simulink model "HeadingControl_DiffDriveRover"  (R2021a)
settings: Solver=ode45  StartTime=0.0  StopTime=15  RelTol=1e-3
values from neighbouring files (symbols this model uses):
  den_motor = [J*L, (J*R + b*L), (b*R + K^2)]    [heading_control_rover.m]
  Kd = 0.8    [heading_control_rover.m]
  Ki = 1.5    [heading_control_rover.m]
  Kp = 5.0    (= 5)    [heading_control_rover.m]
  L_base = 0.30    (= 0.3)    [heading_control_rover.m]
  num_motor = [K]    [heading_control_rover.m]
  r_wheel = 0.05    [heading_control_rover.m]
  Vbase = 1.0    (= 1)    [heading_control_rover.m]
libraries: pid_lib x1
settings Model: Creator=Casto  LastModifiedBy=Casto

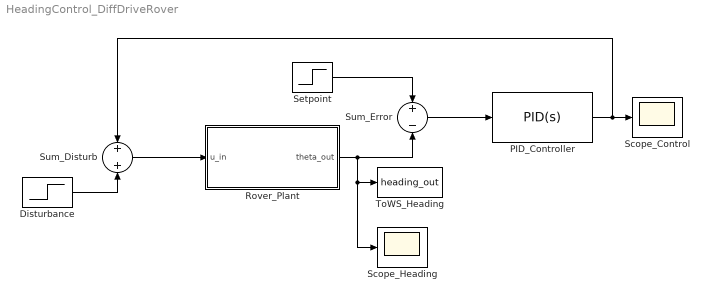
== system HeadingControl_DiffDriveRover ==
  Disturbance : Step  Time=3  After=10  SampleTime=0
  PID_Controller : pid_lib/PID Controller  Controller=PID  Form=Parallel  TimeDomain=Continuous-time  UseExternalTs=off  SampleTime=-1  IntegratorMethod=Forward Euler  FilterMethod=Forward Euler  ControllerParametersSource=internal  P=Kp  I=Ki  D=Kd  UseFilter=on  N=100  TunerSelectOption=Transfer Function Based (PID Tuner App)  InitialConditionSource=internal  InitialConditionForIntegrator=0  InitialConditionForFilter=0  DifferentiatorICPrevScaledInput=0  ExternalReset=none  TrackingMode=off  Kt=1  LimitOutput=off  SatLimitsSource=internal  UpperSaturationLimit=inf  LowerSaturationLimit=-inf  LinearizeAsGain=on  AntiWindupMode=none  Kb=1  POutMin=[]  POutMax=[]  IOutMin=[]  IOutMax=[]  DOutMin=[]  DOutMax=[]  NOutMin=[]  NOutMax=[]  SumOutMin=[]  SumOutMax=[]  SaturationOutMin=[]  SaturationOutMax=[]  PParamMin=[]  PParamMax=[]  IParamMin=[]  IParamMax=[]  DParamMin=[]  DParamMax=[]  NParamMin=[]  NParamMax=[]  KbParamMin=[]  KbParamMax=[]  KtParamMin=[]  KtParamMax=[]  KbOutMin=[]  KbOutMax=[]  KtOutMin=[]  KtOutMax=[]  IntegratorOutMin=[]  IntegratorOutMax=[]  FilterOutMin=[]  FilterOutMax=[]  SumI1OutMin=[]  SumI1OutMax=[]  SumI2OutMin=[]  SumI2OutMax=[]  SumI3OutMin=[]  SumI3OutMax=[]  SumI4OutMin=[]  SumI4OutMax=[]  SumDOutMin=[]  SumDOutMax=[]  DifferentiatorOutMin=[]  DifferentiatorOutMax=[]  FilterDiffOutCoefMin=[]  FilterDiffOutCoefMax=[]  ReciprocalOutMin=[]  ReciprocalOutMax=[]  SumDenOutMin=[]  SumDenOutMax=[]  SumNumOutMin=[]  SumNumOutMax=[]  DivideOutMin=[]  DivideOutMax=[]  UdiffTsProdOutMin=[]  UdiffTsProdOutMax=[]  NTsProdOutMin=[]  NTsProdOutMax=[]  UintegralTsProdOutMin=[]  UintegralTsProdOutMax=[]  UngainTsProdOutMin=[]  UngainTsProdOutMax=[]  IntegratorContinuousStateAttributes=''  IntegratorStateMustResolveToSignalObject=off  IntegratorRTWStateStorageClass=Auto  FilterContinuousStateAttributes=''  FilterStateMustResolveToSignalObject=off  FilterRTWStateStorageClass=Auto  ParallelPVariant=InternalParameters  IdealPVariant=Disabled  IVariant=InternalParameters  DVariant=InternalParameters  IntegratorVariant=Continuous  SatVariant=Disabled  AWVariant=Passthrough  PCopyVariant=Disabled  TRVariant=Disabled  FdbkBlocksVariant=Forward  IdealPFdbkVariant=Disabled  SatFdbkVariant=Disabled  DerivativeFilterVariant=ContFilter  NVariant=InternalParameters  NCopyVariant=Disabled  FilterICVariant=InternalICsFilter  IntegratorICVariant=InternalICs  ExternalResetVariant=Disabled  TRSumVariant=Passthrough  SumFdbkVariant=Disabled  SumVariant=Sum_PID  TsampFilterVariant=InternalTs  TsampNgainVariant=Passthrough  TsampIntegralVariant=Passthrough  ExternalSaturationOutDataTypeStr=Inherit: Same as second input
  Rover_Plant : Subsystem
  Scope_Control : Scope
  Scope_Heading : Scope
  Setpoint : Step  Time=0  After=0  SampleTime=0
  Sum_Disturb : Sum
  Sum_Error : Sum  Inputs=+-
  ToWS_Heading : ToWorkspace  VariableName=heading_out  SampleTime=-1
  wires:
  PID_Controller/1 -> Sum_Disturb/1, Scope_Control/1
  Sum_Error/1 -> PID_Controller/1
  Sum_Disturb/1 -> Rover_Plant/1(u_in)
  Setpoint/1 -> Sum_Error/1
  Disturbance/1 -> Sum_Disturb/2
  Rover_Plant/1(theta_out) -> ToWS_Heading/1, Scope_Heading/1, Sum_Error/2

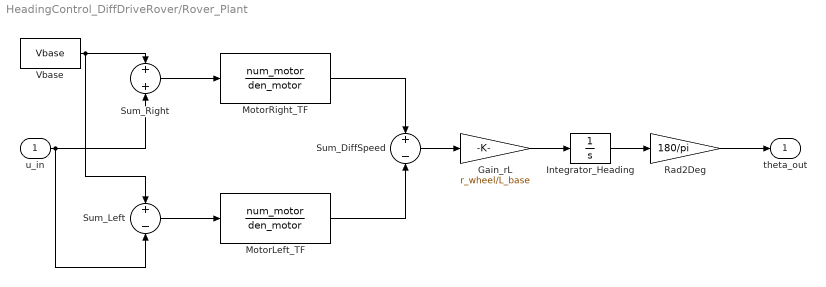
== system HeadingControl_DiffDriveRover/Rover_Plant ==
  u_in : Inport
  Gain_rL : Gain  Gain=r_wheel/L_base
  Integrator_Heading : Integrator
  MotorLeft_TF : TransferFcn  Numerator=num_motor  Denominator=den_motor
  MotorRight_TF : TransferFcn  Numerator=num_motor  Denominator=den_motor
  Rad2Deg : Gain  Gain=180/pi
  Sum_DiffSpeed : Sum  Inputs=+-
  Sum_Left : Sum  Inputs=+-
  Sum_Right : Sum
  Vbase : Constant  Value=Vbase
  theta_out : Outport
  wires:
  u_in/1 -> Sum_Right/2, Sum_Left/2
  Vbase/1 -> Sum_Right/1, Sum_Left/1
  Sum_Right/1 -> MotorRight_TF/1
  Sum_Left/1 -> MotorLeft_TF/1
  MotorRight_TF/1 -> Sum_DiffSpeed/1
  MotorLeft_TF/1 -> Sum_DiffSpeed/2
  Sum_DiffSpeed/1 -> Gain_rL/1
  Gain_rL/1 -> Integrator_Heading/1
  Integrator_Heading/1 -> Rad2Deg/1
  Rad2Deg/1 -> theta_out/1
